simulink model "pythonTestingSimulink"  (R2022b)
settings: Solver=VariableStepAuto  StartTime=0.0  StopTime=10.0  RelTol=1e-3
settings Model: Creator=Ceribro  LastModifiedBy=Ceribro

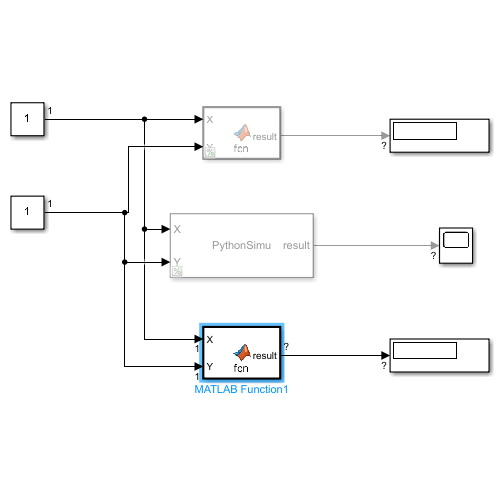
[thumbnail: Simulink's stored preview of the top-level diagram]
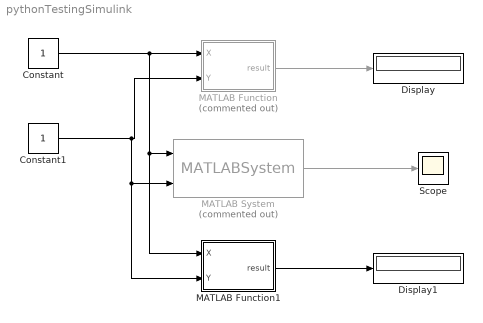
== system pythonTestingSimulink ==
  Constant : Constant
  Constant1 : Constant
  Display : Display
  Display1 : Display
  MATLAB Function : MATLAB Function  Commented=on  TreatAsAtomicUnit=on
  MATLAB Function1 : MATLAB Function  TreatAsAtomicUnit=on
  MATLAB System : MATLABSystem  Commented=on  System=PythonSimu  SimulateUsing=Interpreted execution
      mask Type: PythonSimu
      mask Display:
      | disp('PythonSimu');
      | port_label('input',1,'X');
      | port_label('input',2,'Y');
      | port_label('output',1,'result');
  Scope : Scope
  wires:
  Constant/1 -> MATLAB Function1/1(X), MATLAB System/1, MATLAB Function/1(X)
  Constant1/1 -> MATLAB Function1/2(Y), MATLAB System/2, MATLAB Function/2(Y)
  MATLAB System/1 -> Scope/1
  MATLAB Function/1(result) -> Display/1
  MATLAB Function1/1(result) -> Display1/1

== matlab function pythonTestingSimulink/MATLAB Function ==
  data: X input; result output; Y input
function result = fcn(X,Y)

result=pyrunfile("Matlab_function.py ","z",x=X,y=Y);

== matlab function pythonTestingSimulink/MATLAB Function1 ==
  data: X input; result output; Y input
function result = fcn(X,Y)

result= py.math.sqrt(X)*py.int(Y);
